simulink model "multi__micro1primarysecondarynn"  (R2015a)
settings: Solver=ode23tb  StartTime=0.0  StopTime=2
model workspace: external: MAT-File D:\google drive\project\nn1\matla.mat (data not in the file)
undefined symbols (not defined in the file): cf, gam, gamp, k1, k2, k3, k5, Lc, lf, mp1, mp2, Mu, nq1, nq2, rc, sig, sigp, td, wn
libraries: powerlib x115, powerlib_meascontrol x32, powerlib_extras x2
(part 2 of 3)

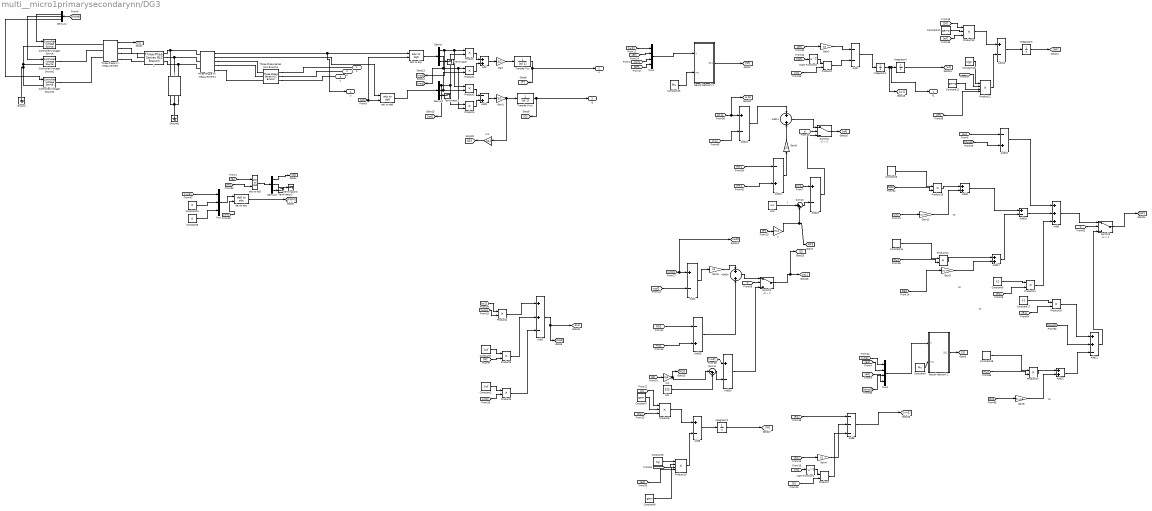
== system multi__micro1primarysecondarynn/DG3 ==
  note: SE
  note: SE
  note: SE
  note: SE
  Add{,3,11,14,17,22} (6 alike) : Sum
  Add{1,13,15..16} (4 alike) : Sum  Inputs=-+
  Add{4,9..10,12,18,20,23} (7 alike) : Sum  Inputs=+-
  Add2 : Sum  Inputs=++-
  Add21 : Sum  Inputs=++-
  Add5 : Sum  Inputs=+++
  Add7 : Sum  Inputs=--
  Add8 : Sum  Inputs=---
  C : powerlib/Elements/Three-Phase Series RLC Branch  LConnTagsString=A|B|C  RConnTagsString=A|B|C  BranchType=C  Resistance=1  Inductance=1e-3  Capacitance=cf  Measurements=None
  Constant1 : Constant  Value=1/cf
  Constant10 : Constant  Value=0
  Constant11 : Constant  Value=gamp
  Constant12 : Constant  Value=gamp
  Constant13 : Constant  Value=sigp
  Constant14 : Constant  Value=-31.446
  Constant15 : Constant  Value=Mu
  Constant17 : Constant  Value=k1
  Constant18 : Constant  Value=-31.446
  Constant2 : Constant  Value=1/cf
  Constant3 : Constant  Value=-31.446
  Constant4 : Constant  Value=Mu
  Constant5 : Constant  Value=k1
  Constant6 : Constant  Value=0
  Constant7 : Constant  Value=gam
  Constant8 : Constant  Value=sig
  Constant9 : Constant  Value=gam
  Controlled Voltage Source : powerlib/Electrical Sources/Controlled Voltage Source  Initialize=on  Source_Type=AC  Amplitude=0  Phase=0  Frequency=0  Measurements=None
  Controlled Voltage Source1 : powerlib/Electrical Sources/Controlled Voltage Source  Initialize=on  Source_Type=AC  Amplitude=0  Phase=0  Frequency=0  Measurements=None
  Controlled Voltage Source2 : powerlib/Electrical Sources/Controlled Voltage Source  Initialize=on  Source_Type=AC  Amplitude=0  Phase=0  Frequency=0  Measurements=None
  Demux{,1,3..4} (4 alike) : Demux  Outputs=3
  Gain : Gain  Gain=3/2
  Gain1 : Gain  Gain=3/2
  Gain11 : Gain  Gain=31.446
  Gain2 : Gain  Gain=k3
  Gain3 : Gain  Gain=31.446
  Gain4 : Gain  Gain=k2
  Gain5 : Gain  Gain=k5
  Gain6 : Gain  Gain=k5
  Gain8 : Gain  Gain=31.446
  Ground : powerlib/Elements/Ground  LConnTagsString=a
  Ground1 : powerlib/Elements/Ground  LConnTagsString=a
  Integrator1 : Integrator  UpperSaturationLimit=321  LowerSaturationLimit=314.16
  Integrator2 : Integrator  InitialCondition=zeros(16,1)  UpperSaturationLimit=314.16  ZeroCross=off
  Integrator3 : Integrator  InitialCondition=zeros(16,1)  UpperSaturationLimit=314.16  ZeroCross=off
  Integrator4 : Integrator  UpperSaturationLimit=314.16  ZeroCross=off
  L : powerlib/Elements/Three-Phase Series RLC Branch  LConnTagsString=A|B|C  RConnTagsString=A|B|C  BranchType=RL  Resistance=0.1  Inductance=lf  Capacitance=1e-6  Measurements=None
  Math Function1 : Math  Operator=transpose  OutputSignalType=real  SaturateOnIntegerOverflow=on
  Math Function3 : Math  Operator=transpose  OutputSignalType=real  SaturateOnIntegerOverflow=on
  Mux : Mux  Inputs=3
  Mux1 : Mux
  Mux2 : Mux
  Neural Network 1 : MATLAB Function  TreatAsAtomicUnit=on
  Neural Network 2 : MATLAB Function  TreatAsAtomicUnit=on
  Product{,1,3..4} (4 alike) : Product  RndMeth=Zero
  Product10 : Product  Inputs=4
  Product{2,5..6,11,14..17} (8 alike) : Product
  Product12 : Product  Inputs=4
  Product13 : Product  Inputs=3
  Product7 : Product  Multiplication=Matrix(*)
  Product8 : Product  Inputs=3
  Product9 : Product  Multiplication=Matrix(*)
  Sum10 : Sum  Inputs=|+-
  Sum11 : Sum  Inputs=|-+
  Switch2 : Switch  Criteria=u2 > Threshold
  Switch3 : Switch  Criteria=u2 > Threshold
  Switch4 : Switch  Criteria=u2 > Threshold
  Terminator{,1..3} (4 alike) : Terminator
  Three-Phase Series RLC Branch4 : powerlib/Elements/Three-Phase Series RLC Branch  LConnTagsString=A|B|C  RConnTagsString=A|B|C  BranchType=RL  Resistance=rc  Inductance=Lc  Capacitance=1e-6  Measurements=None
  Three-Phase V-I Measurement : powerlib/Measurements/Three-Phase V-I Measurement  VoltageMeasurement=no  SetLabelV=off  LabelV=Vabc  Vpu=off  VpuLL=off  CurrentMeasurement=yes  SetLabelI=off  LabelI=Iabc  Ipu=off  Pbase=100e6  Vbase=500e3  OutputType=Complex  PhasorSimulation=off  PSBequivalent=0
  Three-Phase V-I Measurement1 : powerlib/Measurements/Three-Phase V-I Measurement  VoltageMeasurement=phase-to-ground  SetLabelV=off  LabelV=Vabc  Vpu=off  VpuLL=off  CurrentMeasurement=yes  SetLabelI=off  LabelI=Iabc  Ipu=off  Pbase=100e6  Vbase=500e3  OutputType=Complex  PhasorSimulation=off  PSBequivalent=0
  Transfer Fcn : TransferFcn  Denominator=[td 1]
  Transfer Fcn1 : TransferFcn  Denominator=[td 1]
  Un1 : Constant  Value=325
  Un3 : Constant  Value=wn
  abc to dq0 : powerlib_meascontrol/Transformations/abc to dq0  Alignment=90 degrees behind phase A axis
  abc to dq1 : powerlib_meascontrol/Transformations/abc to dq0  Alignment=90 degrees behind phase A axis
  abc to dq3 : powerlib_meascontrol/Transformations/abc to dq0  Alignment=90 degrees behind phase A axis
  dq0 to abc : powerlib_meascontrol/Transformations/dq0 to abc  Alignment=90 degrees behind phase A axis
  m1 : Gain  Gain=nq1
  m2 : Gain  Gain=nq1
  n : Gain  Gain=mp1
  a : PMIOPort  Tag=PMCPort  Port=1  Side=Right
  b : PMIOPort  Tag=PMCPort  Port=2  Side=Right
  c : PMIOPort  Tag=PMCPort  Port=3  Side=Right
  U : Outport
  P : Outport  Port=2
  Q : Outport  Port=3
  f1 : Outport  Port=4
  tag scope: E3=global, MP3=global, NQ3=global, Q33=global, dv3=global, vod3=global, w13=global
  wires:
  [PWM] -> Demux4/1
  Three-Phase V-I Measurement1/1 -> U/1, abc to dq1/1
  Three-Phase V-I Measurement1/2 -> abc to dq0/1
  Demux/1 -> [vod], Product/1, Product3/1
  Demux1/1 -> [iod], Product/2, Product4/1
  Demux/2 -> [voq], Product1/1, Product4/2
  Demux1/2 -> Product1/2, Product3/2
  Product/1 -> Add/1
  Product1/1 -> Add/2
  Product3/1 -> Add1/1
  Product4/1 -> Add1/2
  [wt] -> abc to dq1/2, abc to dq0/2
  Demux4/1 -> Controlled Voltage Source/1
  Demux4/2 -> Controlled Voltage Source1/1
  Demux4/3 -> Controlled Voltage Source2/1
  Three-Phase V-I Measurement/1 -> [IL]
  Add/1 -> Gain/1
  Gain/1 -> Transfer Fcn/1
  Add1/1 -> Gain1/1
  Gain1/1 -> m1/1, Transfer Fcn1/1
  abc to dq1/1 -> Demux/1
  abc to dq0/1 -> Demux1/1
  [w1] -> Product2/1
  [voq] -> Product2/2
  Product2/1 -> Add2/1
  Constant1/1 -> Product5/1
  [Id] -> Product5/2
  Product5/1 -> Add2/2
  Constant2/1 -> Product6/1
  [iod] -> Product6/2
  Product6/1 -> Add2/3
  Add2/1 -> [dvodi], [dv3]
  Demux/3 -> Terminator/1
  Demux1/3 -> Terminator1/1
  Gain4/1 -> Add8/2
  [e2] -> Gain4/1
  [S] -> Product7/2
  [W] -> Math Function1/1
  Math Function1/1 -> Product7/1
  Product7/1 -> Add8/3
  Add8/1 -> [vn1]
  [IL] -> abc to dq3/1
  Demux3/1 -> [Id]
  Demux3/2 -> Terminator3/1
  [wt] -> abc to dq3/2
  Mux/1 -> dq0 to abc/1
  [wt] -> dq0 to abc/2
  abc to dq3/1 -> Demux3/1
  dq0 to abc/1 -> [PWM]
  Demux3/3 -> Terminator2/1
  [vn1] -> Mux/1
  Constant10/1 -> Mux/2
  Constant6/1 -> Mux/3
  Transfer Fcn/1 -> P/1, [P]
  Transfer Fcn1/1 -> Q/1, [Q]
  [ef] -> Gain2/1
  [Sf] -> Product9/2
  [Wf] -> Math Function3/1
  Math Function3/1 -> Product9/1
  Gain2/1 -> Add7/1
  Product9/1 -> Add7/2
  [w1] -> Mux1/1
  [ef] -> Mux1/2
  [wn] -> Mux1/3
  [MP1] -> Mux1/4
  [w1] -> [w13], Add10/1
  [w12] -> Add10/2
  Add10/1 -> Add11/1
  [MP1] -> Add13/1
  [MP3] -> Add13/2
  Add13/1 -> Gain6/1
  [vod] -> [vod3], Add4/1
  [vod2] -> Add4/2
  Add4/1 -> Gain5/1
  Add15/1 -> Add14/2
  Gain6/1 -> Add11/2
  [NQ1] -> Add15/1
  [NQ3] -> Add15/2
  [e1] -> Add8/1
  Gain5/1 -> Add14/1
  [vod] -> Mux2/1
  [e1] -> Mux2/2
  [e2] -> Mux2/4
  [dvodi] -> Mux2/3
  Constant3/1 -> Product15/1
  [NQ3] -> Product15/2
  Product15/1 -> Add3/1
  [Q33] -> Gain11/1
  Constant14/1 -> Product14/1
  [NQ1] -> Product14/2
  Product14/1 -> Add17/1
  [Q22] -> Gain3/1
  Add17/1 -> Add18/2
  Add3/1 -> Add18/1
  Gain3/1 -> Add17/2
  Gain11/1 -> Add3/2
  Add18/1 -> Add5/2
  Constant5/1 -> Product11/1
  [e1] -> Product11/2
  Product11/1 -> Add5/3
  [dv2] -> Add16/1
  Add16/1 -> Add5/1
  [dvodi] -> Add16/2
  m1/1 -> [Q33]
  Neural Network 1/1(Sz1) -> [Sf]
  Neural Network 2/1(Sz1) -> [S]
  [S] -> Product8/1
  Constant7/1 -> Product8/2
  [e2] -> Product8/3
  Product8/1 -> Add9/1
  Constant8/1 -> Product10/1
  [W] -> Product10/2
  Product10/1 -> Add9/2
  Constant9/1 -> Product10/3
  Add9/1 -> Integrator2/1
  Integrator2/1 -> [W]
  [e2] -> Product10/4
  [Sf] -> Product13/1
  Constant12/1 -> Product13/2
  [ef] -> Product13/3
  Product13/1 -> Add12/1
  Constant13/1 -> Product12/1
  [Wf] -> Product12/2
  Product12/1 -> Add12/2
  Constant11/1 -> Product12/3
  Add12/1 -> Integrator3/1
  Integrator3/1 -> [Wf]
  [ef] -> Product12/4
  Constant4/1 -> Neural Network 2/2(mu)
  Mux2/1 -> Neural Network 2/1(X)
  Constant15/1 -> Neural Network 1/2(mu)
  Mux1/1 -> Neural Network 1/1(X)
  [ti] -> Switch2/2
  Add20/1 -> Switch2/3
  Add14/1 -> Switch2/1
  Switch2/1 -> [E3], [e1]
  [vod] -> Add20/1
  [Q] -> m2/1
  Un1/1 -> Sum11/2
  m2/1 -> [NQ3], Sum11/1
  Sum11/1 -> Add20/2
  [dvodi] -> Add21/2
  Constant17/1 -> Product16/1
  [e1] -> Product16/2
  Product16/1 -> Add21/1
  Constant18/1 -> Product17/1
  [NQ3] -> Product17/2
  Product17/1 -> Add22/1
  [Q33] -> Gain8/1
  Add22/1 -> Add21/3
  Gain8/1 -> Add22/2
  [ti] -> Switch3/2
  Add5/1 -> Switch3/1
  Switch3/1 -> [e2]
  Add21/1 -> Switch3/3
  [P] -> n/1
  Un3/1 -> Sum10/1  "f"
  Sum10/1 -> Add23/2
  n/1 -> [MP3], Sum10/2
  [w1] -> Add23/1
  [ti] -> Switch4/2
  Add11/1 -> Switch4/1
  Switch4/1 -> [ef]
  Add23/1 -> Switch4/3
  Add7/1 -> Integrator1/1
  Integrator4/1 -> [wt]
  Integrator1/1 -> [w1], f1/1, Integrator4/1
  connections:
  C/RConn1 -- Ground1/LConn1 -- C/RConn3 -- C/RConn2
  L/RConn2 -- Three-Phase V-I Measurement1/LConn2 -- C/LConn2
  L/RConn1 -- Three-Phase V-I Measurement1/LConn1 -- C/LConn1
  L/RConn3 -- Three-Phase V-I Measurement1/LConn3 -- C/LConn3
  Controlled Voltage Source/LConn1 -- Controlled Voltage Source1/LConn1 -- Ground/LConn1 -- Controlled Voltage Source2/LConn1
  Three-Phase V-I Measurement/LConn1 -- Controlled Voltage Source/RConn1
  Controlled Voltage Source1/RConn1 -- Three-Phase V-I Measurement/LConn2
  Controlled Voltage Source2/RConn1 -- Three-Phase V-I Measurement/LConn3
  Three-Phase V-I Measurement/RConn1 -- L/LConn1
  Three-Phase V-I Measurement/RConn2 -- L/LConn2
  Three-Phase V-I Measurement/RConn3 -- L/LConn3
  Three-Phase V-I Measurement1/RConn1 -- Three-Phase Series RLC Branch4/RConn1
  Three-Phase V-I Measurement1/RConn2 -- Three-Phase Series RLC Branch4/RConn2
  Three-Phase V-I Measurement1/RConn3 -- Three-Phase Series RLC Branch4/RConn3
  Three-Phase Series RLC Branch4/LConn1 -- a/RConn1
  Three-Phase Series RLC Branch4/LConn2 -- b/RConn1
  Three-Phase Series RLC Branch4/LConn3 -- c/RConn1

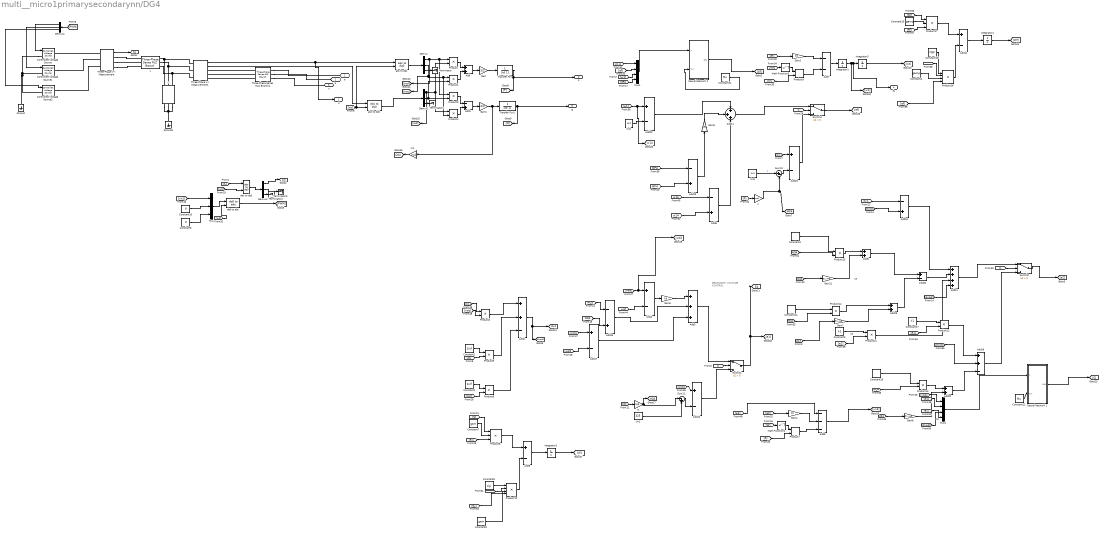
== system multi__micro1primarysecondarynn/DG4 ==
  note: SECONDARY VOLTAGE CONTROL
  note: SE
  note: SE
  note: SE
  Add{,5,19,22} (4 alike) : Sum
  Add{1,6,13,15,18} (5 alike) : Sum  Inputs=-+
  Add{4,9..10,12,14,17,20,23} (8 alike) : Sum  Inputs=+-
  Add11 : Sum  Inputs=+++
  Add16 : Sum  Inputs=++-
  Add2 : Sum  Inputs=++-
  Add21 : Sum  Inputs=++++
  Add3 : Sum  Inputs=+++
  Add7 : Sum  Inputs=--
  Add8 : Sum  Inputs=---
  C : powerlib/Elements/Three-Phase Series RLC Branch  LConnTagsString=A|B|C  RConnTagsString=A|B|C  BranchType=C  Resistance=1  Inductance=1e-3  Capacitance=cf  Measurements=None
  Constant1 : Constant  Value=1/cf
  Constant10 : Constant  Value=0
  Constant11 : Constant  Value=Mu
  Constant12 : Constant  Value=Mu
  Constant14 : Constant  Value=-31.446
  Constant15 : Constant  Value=gamp
  Constant16 : Constant  Value=sigp
  Constant17 : Constant  Value=k1
  Constant18 : Constant  Value=-31.446
  Constant2 : Constant  Value=1/cf
  Constant3 : Constant  Value=-31.446
  Constant4 : Constant  Value=gamp
  Constant5 : Constant  Value=k1
  Constant6 : Constant  Value=0
  Constant7 : Constant  Value=gam
  Constant8 : Constant  Value=sig
  Constant9 : Constant  Value=gam
  Controlled Voltage Source : powerlib/Electrical Sources/Controlled Voltage Source  Initialize=off  Source_Type=AC  Amplitude=325  Phase=0  Frequency=50  Measurements=None
  Controlled Voltage Source1 : powerlib/Electrical Sources/Controlled Voltage Source  Initialize=off  Source_Type=AC  Amplitude=325  Phase=0  Frequency=50  Measurements=None
  Controlled Voltage Source2 : powerlib/Electrical Sources/Controlled Voltage Source  Initialize=off  Source_Type=AC  Amplitude=325  Phase=0  Frequency=50  Measurements=None
  Demux{,1,3..4} (4 alike) : Demux  Outputs=3
  Gain : Gain  Gain=3/2
  Gain1 : Gain  Gain=3/2
  Gain11 : Gain  Gain=31.446
  Gain2 : Gain  Gain=k3
  Gain4 : Gain  Gain=k2
  Gain5 : Gain  Gain=k5
  Gain6 : Gain  Gain=k5
  Gain7 : Gain  Gain=31.446
  Gain8 : Gain  Gain=31.446
  Ground : powerlib/Elements/Ground  LConnTagsString=a
  Ground1 : powerlib/Elements/Ground  LConnTagsString=a
  Integrator1 : Integrator  UpperSaturationLimit=321  LowerSaturationLimit=314.16
  Integrator2 : Integrator  InitialCondition=zeros(16,1)  UpperSaturationLimit=314.16  ZeroCross=off
  Integrator3 : Integrator  UpperSaturationLimit=314.16  ZeroCross=off
  Integrator4 : Integrator  InitialCondition=zeros(16,1)  UpperSaturationLimit=314.16  ZeroCross=off
  L : powerlib/Elements/Three-Phase Series RLC Branch  LConnTagsString=A|B|C  RConnTagsString=A|B|C  BranchType=RL  Resistance=0.1  Inductance=lf  Capacitance=1e-6  Measurements=None
  Math Function1 : Math  Operator=transpose  OutputSignalType=real  SaturateOnIntegerOverflow=on
  Math Function3 : Math  Operator=transpose  OutputSignalType=real  SaturateOnIntegerOverflow=on
  Mux : Mux  Inputs=3
  Mux1 : Mux
  Mux2 : Mux
  Neural Network 1 : MATLAB Function  TreatAsAtomicUnit=on
  Neural Network 2 : MATLAB Function  TreatAsAtomicUnit=on
  Product{,1,3..4} (4 alike) : Product  RndMeth=Zero
  Product10 : Product  Inputs=4
  Product{2,5..6,11..15} (8 alike) : Product
  Product16 : Product  Inputs=4
  Product17 : Product  Inputs=3
  Product7 : Product  Multiplication=Matrix(*)
  Product8 : Product  Inputs=3
  Product9 : Product  Multiplication=Matrix(*)
  Sum10 : Sum  Inputs=|+-
  Sum11 : Sum  Inputs=|-+
  Switch2 : Switch  Criteria=u2 > Threshold
  Switch3 : Switch  Criteria=u2 > Threshold
  Switch4 : Switch  Criteria=u2 > Threshold
  Terminator{,1..3} (4 alike) : Terminator
  Three-Phase Series RLC Branch4 : powerlib/Elements/Three-Phase Series RLC Branch  LConnTagsString=A|B|C  RConnTagsString=A|B|C  BranchType=RL  Resistance=rc  Inductance=Lc  Capacitance=1e-6  Measurements=None
  Three-Phase V-I Measurement : powerlib/Measurements/Three-Phase V-I Measurement  VoltageMeasurement=no  SetLabelV=off  LabelV=Vabc  Vpu=off  VpuLL=off  CurrentMeasurement=yes  SetLabelI=off  LabelI=Iabc  Ipu=off  Pbase=100e6  Vbase=500e3  OutputType=Complex  PhasorSimulation=off  PSBequivalent=0
  Three-Phase V-I Measurement1 : powerlib/Measurements/Three-Phase V-I Measurement  VoltageMeasurement=phase-to-ground  SetLabelV=off  LabelV=Vabc  Vpu=off  VpuLL=off  CurrentMeasurement=yes  SetLabelI=off  LabelI=Iabc  Ipu=off  Pbase=100e6  Vbase=500e3  OutputType=Complex  PhasorSimulation=off  PSBequivalent=0
  Transfer Fcn : TransferFcn  Denominator=[td 1]
  Transfer Fcn1 : TransferFcn  Denominator=[td 1]
  Un1 : Constant  Value=325
  Un2 : Constant  Value=wn
  Un3 : Constant  Value=wn
  abc to dq0 : powerlib_meascontrol/Transformations/abc to dq0  Alignment=90 degrees behind phase A axis
  abc to dq1 : powerlib_meascontrol/Transformations/abc to dq0  Alignment=90 degrees behind phase A axis
  abc to dq3 : powerlib_meascontrol/Transformations/abc to dq0  Alignment=90 degrees behind phase A axis
  dq0 to abc : powerlib_meascontrol/Transformations/dq0 to abc  Alignment=90 degrees behind phase A axis
  m : Gain  Gain=nq1
  m1 : Gain  Gain=nq1
  n : Gain  Gain=mp1
  a : PMIOPort  Tag=PMCPort  Port=1  Side=Right
  b : PMIOPort  Tag=PMCPort  Port=2  Side=Right
  c : PMIOPort  Tag=PMCPort  Port=3  Side=Right
  U : Outport
  P : Outport  Port=2
  Q : Outport  Port=3
  f1 : Outport  Port=4
  tag scope: E4=global, MP4=global, NQ4=global, Q44=global, dv4=global, vod4=global, w14=global
  wires:
  [PWM] -> Demux4/1
  Three-Phase V-I Measurement1/1 -> U/1, abc to dq1/1
  Demux/1 -> [vod], Product/1, Product3/1
  Demux1/1 -> [iod], Product/2, Product4/1
  Demux/2 -> [voq], Product1/1, Product4/2
  Demux1/2 -> Product1/2, Product3/2
  Product/1 -> Add/1
  Product1/1 -> Add/2
  Product3/1 -> Add1/1
  Product4/1 -> Add1/2
  [wt] -> abc to dq1/2, abc to dq0/2
  Demux4/1 -> Controlled Voltage Source/1
  Demux4/2 -> Controlled Voltage Source1/1
  Demux4/3 -> Controlled Voltage Source2/1
  Three-Phase V-I Measurement/1 -> [IL]
  Add/1 -> Gain/1
  Gain/1 -> Transfer Fcn/1
  Add1/1 -> Gain1/1
  Gain1/1 -> m1/1, Transfer Fcn1/1
  abc to dq1/1 -> Demux/1
  abc to dq0/1 -> Demux1/1
  [w1] -> Product2/1
  [voq] -> Product2/2
  Product2/1 -> Add2/1
  Constant1/1 -> Product5/1
  [Id] -> Product5/2
  Product5/1 -> Add2/2
  Constant2/1 -> Product6/1
  [iod] -> Product6/2
  Product6/1 -> Add2/3
  Add2/1 -> [dvodi], [dv4]
  Demux/3 -> Terminator/1
  Demux1/3 -> Terminator1/1
  [vod] -> [vod4], Add4/1
  Gain4/1 -> Add8/2
  [e2] -> Gain4/1
  [S] -> Product7/2
  [W] -> Math Function1/1
  Math Function1/1 -> Product7/1
  Product7/1 -> Add8/3
  [vref] -> Add4/2
  Add8/1 -> [vn1]
  [IL] -> abc to dq3/1
  Demux3/1 -> [Id]
  Demux3/2 -> Terminator3/1
  [wt] -> abc to dq3/2
  Mux/1 -> dq0 to abc/1
  [wt] -> dq0 to abc/2
  abc to dq3/1 -> Demux3/1
  dq0 to abc/1 -> [PWM]
  Demux3/3 -> Terminator2/1
  [vn1] -> Mux/1
  Constant10/1 -> Mux/2
  Constant6/1 -> Mux/3
  Transfer Fcn/1 -> P/1, [P]
  Transfer Fcn1/1 -> Q/1, [Q]
  [w1] -> Mux1/1
  [ef] -> Mux1/2
  [w1] -> Mux1/3
  [MP2] -> Mux1/4
  [ef] -> Gain2/1
  [Sf] -> Product9/2
  [Wf] -> Math Function3/1
  Math Function3/1 -> Product9/1
  Gain2/1 -> Add7/1
  Product9/1 -> Add7/2
  [w1] -> [w14], Add10/1
  Un2/1 -> Add10/2
  Add10/1 -> Add11/1
  Three-Phase V-I Measurement1/2 -> abc to dq0/1
  [MP3] -> Add13/1
  [MP4] -> Add13/2
  Add13/1 -> Gain6/1
  Gain6/1 -> Add11/2
  [NQ3] -> Add15/1
  [NQ4] -> Add15/2
  [e1] -> Add8/1
  Add4/1 -> Gain5/1
  Gain5/1 -> Add3/1
  Add15/1 -> Add3/2
  [vod3] -> Add17/2
  [vod] -> Add17/1
  Add17/1 -> Add3/3
  Constant3/1 -> Product15/1
  [NQ4] -> Product15/2
  Product15/1 -> Add5/1
  [Q44] -> Gain11/1
  Constant14/1 -> Product14/1
  [NQ3] -> Product14/2
  Product14/1 -> Add19/1
  [Q33] -> Gain7/1
  Add19/1 -> Add20/2
  Add5/1 -> Add20/1
  Gain7/1 -> Add19/2
  Gain11/1 -> Add5/2
  Add20/1 -> Add21/2
  Constant5/1 -> Product11/1
  [e1] -> Product11/2
  Product11/1 -> Add21/3
  [dv3] -> Add18/1
  Add18/1 -> Add21/1
  [dvodi] -> Add18/2
  [vod] -> Mux2/1
  [e1] -> Mux2/2
  [e2] -> Mux2/4
  [dvodi] -> Mux2/3
  [dvodi] -> Add21/4
  m1/1 -> [Q44]
  [w13] -> Add6/1
  [w14] -> Add6/2
  Add6/1 -> Add11/3
  [S] -> Product8/1
  Constant7/1 -> Product8/2
  [e2] -> Product8/3
  Product8/1 -> Add9/1
  Constant8/1 -> Product10/1
  [W] -> Product10/2
  Product10/1 -> Add9/2
  Constant9/1 -> Product10/3
  Add9/1 -> Integrator2/1
  Integrator2/1 -> [W]
  [e2] -> Product10/4
  [Sf] -> Product17/1
  Constant15/1 -> Product17/2
  [ef] -> Product17/3
  Product17/1 -> Add14/1
  Constant16/1 -> Product16/1
  [Wf] -> Product16/2
  Product16/1 -> Add14/2
  Constant4/1 -> Product16/3
  Add14/1 -> Integrator4/1
  Integrator4/1 -> [Wf]
  [ef] -> Product16/4
  Neural Network 2/1(Sz1) -> [Sf]
  Constant11/1 -> Neural Network 2/2(mu)
  Mux1/1 -> Neural Network 2/1(X)
  Neural Network 1/1(Sz1) -> [S]
  Constant12/1 -> Neural Network 1/2(mu)
  Mux2/1 -> Neural Network 1/1(X)
  [vod] -> Add12/1
  [Q] -> m/1
  Un1/1 -> Sum11/2
  m/1 -> [NQ4], Sum11/1
  Sum11/1 -> Add12/2
  [ti] -> Switch2/2
  Add12/1 -> Switch2/3
  Add3/1 -> Switch2/1
  Switch2/1 -> [E4], [e1]
  [dvodi] -> Add16/2
  Constant17/1 -> Product12/1
  [e1] -> Product12/2
  Product12/1 -> Add16/1
  Constant18/1 -> Product13/1
  [NQ4] -> Product13/2
  Product13/1 -> Add22/1
  [Q44] -> Gain8/1
  Add22/1 -> Add16/3
  Gain8/1 -> Add22/2
  [ti] -> Switch3/2
  Switch3/1 -> [e2]
  Add21/1 -> Switch3/1
  Add16/1 -> Switch3/3
  Add7/1 -> Integrator1/1
  Integrator3/1 -> [wt]
  Integrator1/1 -> [w1], f1/1, Integrator3/1
  [ti] -> Switch4/2
  Add11/1 -> Switch4/1
  Switch4/1 -> [ef]
  [P] -> n/1
  Un3/1 -> Sum10/1  "f"
  Sum10/1 -> Add23/2
  n/1 -> [MP4], Sum10/2
  [w1] -> Add23/1
  Add23/1 -> Switch4/3
  connections:
  C/RConn1 -- Ground1/LConn1 -- C/RConn3 -- C/RConn2
  L/RConn2 -- Three-Phase V-I Measurement1/LConn2 -- C/LConn2
  L/RConn1 -- Three-Phase V-I Measurement1/LConn1 -- C/LConn1
  L/RConn3 -- Three-Phase V-I Measurement1/LConn3 -- C/LConn3
  Controlled Voltage Source/LConn1 -- Controlled Voltage Source1/LConn1 -- Ground/LConn1 -- Controlled Voltage Source2/LConn1
  Three-Phase V-I Measurement/LConn1 -- Controlled Voltage Source/RConn1
  Controlled Voltage Source1/RConn1 -- Three-Phase V-I Measurement/LConn2
  Controlled Voltage Source2/RConn1 -- Three-Phase V-I Measurement/LConn3
  Three-Phase V-I Measurement/RConn1 -- L/LConn1
  Three-Phase V-I Measurement/RConn2 -- L/LConn2
  Three-Phase V-I Measurement/RConn3 -- L/LConn3
  Three-Phase Series RLC Branch4/RConn1 -- Three-Phase V-I Measurement1/RConn1
  Three-Phase Series RLC Branch4/RConn2 -- Three-Phase V-I Measurement1/RConn2
  Three-Phase Series RLC Branch4/RConn3 -- Three-Phase V-I Measurement1/RConn3
  Three-Phase Series RLC Branch4/LConn3 -- c/RConn1
  Three-Phase Series RLC Branch4/LConn2 -- b/RConn1
  Three-Phase Series RLC Branch4/LConn1 -- a/RConn1

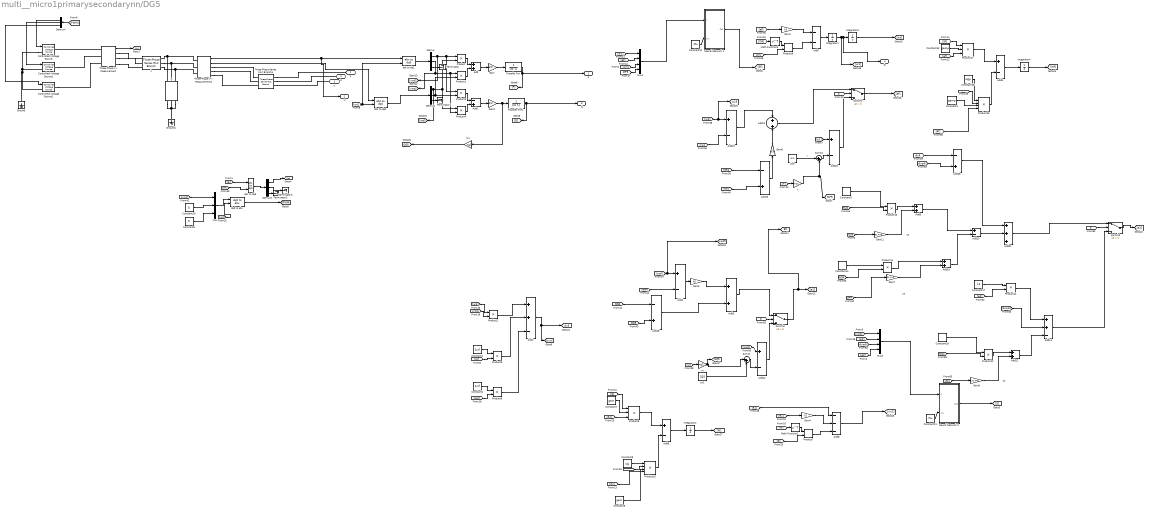
== system multi__micro1primarysecondarynn/DG5 ==
  note: SE
  note: SE
  note: SE
  Add{,3,5,11,19,22} (6 alike) : Sum
  Add{1,13,15,18} (4 alike) : Sum  Inputs=-+
  Add{4,6,9..10,12,20,23} (7 alike) : Sum  Inputs=+-
  Add14 : Sum  Inputs=++-
  Add2 : Sum  Inputs=++-
  Add21 : Sum  Inputs=+++
  Add7 : Sum  Inputs=--
  Add8 : Sum  Inputs=---
  C : powerlib/Elements/Three-Phase Series RLC Branch  LConnTagsString=A|B|C  RConnTagsString=A|B|C  BranchType=C  Resistance=1  Inductance=1e-3  Capacitance=cf  Measurements=None
  Constant1 : Constant  Value=1/cf
  Constant10 : Constant  Value=0
  Constant11 : Constant  Value=Mu
  Constant12 : Constant  Value=Mu
  Constant14 : Constant  Value=-31.446
  Constant15 : Constant  Value=gamp
  Constant16 : Constant  Value=sigp
  Constant17 : Constant  Value=k1
  Constant18 : Constant  Value=-31.446
  Constant2 : Constant  Value=1/cf
  Constant3 : Constant  Value=-31.446
  Constant4 : Constant  Value=gamp
  Constant6 : Constant  Value=0
  Constant7 : Constant  Value=gam
  Constant8 : Constant  Value=sig
  Constant9 : Constant  Value=gam
  Controlled Voltage Source : powerlib/Electrical Sources/Controlled Voltage Source  Initialize=off  Source_Type=AC  Amplitude=325  Phase=0  Frequency=50  Measurements=None
  Controlled Voltage Source1 : powerlib/Electrical Sources/Controlled Voltage Source  Initialize=off  Source_Type=AC  Amplitude=325  Phase=0  Frequency=50  Measurements=None
  Controlled Voltage Source2 : powerlib/Electrical Sources/Controlled Voltage Source  Initialize=off  Source_Type=AC  Amplitude=325  Phase=0  Frequency=50  Measurements=None
  Demux{,1,3..4} (4 alike) : Demux  Outputs=3
  Gain : Gain  Gain=3/2
  Gain1 : Gain  Gain=3/2
  Gain11 : Gain  Gain=31.446
  Gain2 : Gain  Gain=k3
  Gain4 : Gain  Gain=k2
  Gain5 : Gain  Gain=k5
  Gain6 : Gain  Gain=k5
  Gain7 : Gain  Gain=31.446
  Gain8 : Gain  Gain=31.446
  Ground : powerlib/Elements/Ground  LConnTagsString=a
  Ground1 : powerlib/Elements/Ground  LConnTagsString=a
  Integrator1 : Integrator  UpperSaturationLimit=321  LowerSaturationLimit=314.16
  Integrator2 : Integrator  InitialCondition=zeros(16,1)  UpperSaturationLimit=314.16  ZeroCross=off
  Integrator3 : Integrator  UpperSaturationLimit=314.16  ZeroCross=off
  Integrator4 : Integrator  InitialCondition=zeros(16,1)  UpperSaturationLimit=314.16  ZeroCross=off
  L : powerlib/Elements/Three-Phase Series RLC Branch  LConnTagsString=A|B|C  RConnTagsString=A|B|C  BranchType=RL  Resistance=0.1  Inductance=lf  Capacitance=1e-6  Measurements=None
  Math Function1 : Math  Operator=transpose  OutputSignalType=real  SaturateOnIntegerOverflow=on
  Math Function3 : Math  Operator=transpose  OutputSignalType=real  SaturateOnIntegerOverflow=on
  Mux : Mux  Inputs=3
  Mux1 : Mux
  Mux2 : Mux
  Neural Network 1 : MATLAB Function  TreatAsAtomicUnit=on
  Neural Network 2 : MATLAB Function  TreatAsAtomicUnit=on
  Product{,1,3..4} (4 alike) : Product  RndMeth=Zero
  Product10 : Product  Inputs=4
  Product{2,5..6,11..12,14..15} (7 alike) : Product
  Product16 : Product  Inputs=4
  Product17 : Product  Inputs=3
  Product7 : Product  Multiplication=Matrix(*)
  Product8 : Product  Inputs=3
  Product9 : Product  Multiplication=Matrix(*)
  Sum10 : Sum  Inputs=|+-
  Sum11 : Sum  Inputs=|-+
  Switch2 : Switch  Criteria=u2 > Threshold
  Switch3 : Switch  Criteria=u2 > Threshold
  Switch4 : Switch  Criteria=u2 > Threshold
  Terminator{,1..3} (4 alike) : Terminator
  Three-Phase Series RLC Branch4 : powerlib/Elements/Three-Phase Series RLC Branch  LConnTagsString=A|B|C  RConnTagsString=A|B|C  BranchType=RL  Resistance=rc  Inductance=Lc  Capacitance=1e-6  Measurements=None
  Three-Phase V-I Measurement : powerlib/Measurements/Three-Phase V-I Measurement  VoltageMeasurement=no  SetLabelV=off  LabelV=Vabc  Vpu=off  VpuLL=off  CurrentMeasurement=yes  SetLabelI=off  LabelI=Iabc  Ipu=off  Pbase=100e6  Vbase=500e3  OutputType=Complex  PhasorSimulation=off  PSBequivalent=0
  Three-Phase V-I Measurement1 : powerlib/Measurements/Three-Phase V-I Measurement  VoltageMeasurement=phase-to-ground  SetLabelV=off  LabelV=Vabc  Vpu=off  VpuLL=off  CurrentMeasurement=yes  SetLabelI=off  LabelI=Iabc  Ipu=off  Pbase=100e6  Vbase=500e3  OutputType=Complex  PhasorSimulation=off  PSBequivalent=0
  Transfer Fcn : TransferFcn  Denominator=[td 1]
  Transfer Fcn1 : TransferFcn  Denominator=[td 1]
  Un1 : Constant  Value=325
  Un3 : Constant  Value=wn
  abc to dq0 : powerlib_meascontrol/Transformations/abc to dq0  Alignment=90 degrees behind phase A axis
  abc to dq1 : powerlib_meascontrol/Transformations/abc to dq0  Alignment=90 degrees behind phase A axis
  abc to dq3 : powerlib_meascontrol/Transformations/abc to dq0  Alignment=90 degrees behind phase A axis
  dq0 to abc : powerlib_meascontrol/Transformations/dq0 to abc  Alignment=90 degrees behind phase A axis
  m : Gain  Gain=nq1
  m1 : Gain  Gain=nq1
  n : Gain  Gain=mp1
  a : PMIOPort  Tag=PMCPort  Port=1  Side=Right
  b : PMIOPort  Tag=PMCPort  Port=2  Side=Right
  c : PMIOPort  Tag=PMCPort  Port=3  Side=Right
  U : Outport
  P : Outport  Port=2
  Q : Outport  Port=3
  f1 : Outport  Port=4
  tag scope: E5=global, MP5=global, NQ5=global, Q55=global, dv5=global, vod5=global, w15=global
  wires:
  [PWM] -> Demux4/1
  Three-Phase V-I Measurement1/1 -> U/1, abc to dq1/1
  Three-Phase V-I Measurement1/2 -> abc to dq0/1
  Demux/1 -> [vod], Product/1, Product3/1
  Demux1/1 -> [iod], Product/2, Product4/1
  Demux/2 -> [voq], Product1/1, Product4/2
  Demux1/2 -> Product1/2, Product3/2
  Product/1 -> Add/1
  Product1/1 -> Add/2
  Product3/1 -> Add1/1
  Product4/1 -> Add1/2
  [wt] -> abc to dq1/2, abc to dq0/2
  Demux4/1 -> Controlled Voltage Source/1
  Demux4/2 -> Controlled Voltage Source1/1
  Demux4/3 -> Controlled Voltage Source2/1
  Three-Phase V-I Measurement/1 -> [IL]
  Add/1 -> Gain/1
  Gain/1 -> Transfer Fcn/1
  Add1/1 -> Gain1/1
  Gain1/1 -> m1/1, Transfer Fcn1/1
  abc to dq1/1 -> Demux/1
  abc to dq0/1 -> Demux1/1
  [w1] -> Product2/1
  [voq] -> Product2/2
  Product2/1 -> Add2/1
  Constant1/1 -> Product5/1
  [Id] -> Product5/2
  Product5/1 -> Add2/2
  Constant2/1 -> Product6/1
  [iod] -> Product6/2
  Product6/1 -> Add2/3
  Add2/1 -> [dvodi], [dv5]
  Demux/3 -> Terminator/1
  Demux1/3 -> Terminator1/1
  Gain4/1 -> Add8/2
  [e2] -> Gain4/1
  [S] -> Product7/2
  [W] -> Math Function1/1
  Math Function1/1 -> Product7/1
  Product7/1 -> Add8/3
  Add8/1 -> [vn1]
  [IL] -> abc to dq3/1
  Demux3/1 -> [Id]
  Demux3/2 -> Terminator3/1
  [wt] -> abc to dq3/2
  Mux/1 -> dq0 to abc/1
  [wt] -> dq0 to abc/2
  abc to dq3/1 -> Demux3/1
  dq0 to abc/1 -> [PWM]
  Demux3/3 -> Terminator2/1
  [vn1] -> Mux/1
  Constant10/1 -> Mux/2
  Constant6/1 -> Mux/3
  Transfer Fcn/1 -> P/1, [P]
  Transfer Fcn1/1 -> Q/1, [Q]
  [ef] -> Gain2/1
  [Sf] -> Product9/2
  [Wf] -> Math Function3/1
  Math Function3/1 -> Product9/1
  Gain2/1 -> Add7/1
  Product9/1 -> Add7/2
  [w1] -> Mux1/1
  [ef] -> Mux1/2
  [wn] -> Mux1/3
  [MP5] -> Mux1/4
  [w1] -> [w15], Add10/1
  [w14] -> Add10/2
  Add10/1 -> Add11/1
  [MP4] -> Add13/1
  [MP5] -> Add13/2
  Add13/1 -> Gain6/1
  [vod] -> [vod5], Add4/1
  [vod4] -> Add4/2
  Gain6/1 -> Add11/2
  [NQ4] -> Add15/1
  [NQ5] -> Add15/2
  [e1] -> Add8/1
  Add4/1 -> Gain5/1
  Add15/1 -> Add3/2
  Gain5/1 -> Add3/1
  Constant3/1 -> Product15/1
  [NQ5] -> Product15/2
  Product15/1 -> Add5/1
  [Q55] -> Gain11/1
  Constant14/1 -> Product14/1
  [NQ4] -> Product14/2
  Product14/1 -> Add19/1
  [Q44] -> Gain7/1
  Add19/1 -> Add20/2
  Add5/1 -> Add20/1
  Gain7/1 -> Add19/2
  Gain11/1 -> Add5/2
  Add20/1 -> Add21/2
  [dv4] -> Add18/1
  Add18/1 -> Add21/1
  [dvodi] -> Add18/2
  [vod] -> Mux2/1
  [e1] -> Mux2/2
  [e2] -> Mux2/4
  [dvodi] -> Mux2/3
  m1/1 -> [Q55]
  Neural Network 2/1(Sz1) -> [S]
  Neural Network 1/1(Sz1) -> [Sf]
  [S] -> Product8/1
  Constant7/1 -> Product8/2
  [e2] -> Product8/3
  Product8/1 -> Add9/1
  Constant8/1 -> Product10/1
  [W] -> Product10/2
  Product10/1 -> Add9/2
  Constant9/1 -> Product10/3
  Add9/1 -> Integrator2/1
  Integrator2/1 -> [W]
  [e2] -> Product10/4
  [Sf] -> Product17/1
  Constant15/1 -> Product17/2
  [ef] -> Product17/3
  Product17/1 -> Add6/1
  Constant16/1 -> Product16/1
  [Wf] -> Product16/2
  Product16/1 -> Add6/2
  Constant4/1 -> Product16/3
  Add6/1 -> Integrator4/1
  Integrator4/1 -> [Wf]
  [ef] -> Product16/4
  Constant11/1 -> Neural Network 2/2(mu)
  Mux2/1 -> Neural Network 2/1(X)
  Constant12/1 -> Neural Network 1/2(mu)
  Mux1/1 -> Neural Network 1/1(X)
  [ti] -> Switch4/2
  Add11/1 -> Switch4/1
  Switch4/1 -> [ef]
  [P] -> n/1
  Un3/1 -> Sum10/1  "f"
  Sum10/1 -> Add23/2
  n/1 -> [MP5], Sum10/2
  [w1] -> Add23/1
  Add23/1 -> Switch4/3
  Add7/1 -> Integrator1/1
  Integrator3/1 -> [wt]
  Integrator1/1 -> [w1], f1/1, Integrator3/1
  [ti] -> Switch2/2
  Add12/1 -> Switch2/3
  Add3/1 -> Switch2/1
  Switch2/1 -> [E5], [e1]
  [vod] -> Add12/1
  [Q] -> m/1
  Un1/1 -> Sum11/2
  m/1 -> [NQ5], Sum11/1
  Sum11/1 -> Add12/2
  [dvodi] -> Add14/2
  Constant17/1 -> Product11/1
  [e1] -> Product11/2
  Product11/1 -> Add14/1
  Constant18/1 -> Product12/1
  [NQ5] -> Product12/2
  Product12/1 -> Add22/1
  [Q55] -> Gain8/1
  Add22/1 -> Add14/3
  Gain8/1 -> Add22/2
  [ti] -> Switch3/2
  Switch3/1 -> [e2]
  Add21/1 -> Switch3/1
  Add14/1 -> Switch3/3
  connections:
  C/RConn1 -- Ground1/LConn1 -- C/RConn3 -- C/RConn2
  L/RConn2 -- Three-Phase V-I Measurement1/LConn2 -- C/LConn2
  L/RConn1 -- Three-Phase V-I Measurement1/LConn1 -- C/LConn1
  L/RConn3 -- Three-Phase V-I Measurement1/LConn3 -- C/LConn3
  Controlled Voltage Source/LConn1 -- Controlled Voltage Source1/LConn1 -- Ground/LConn1 -- Controlled Voltage Source2/LConn1
  Three-Phase V-I Measurement/LConn1 -- Controlled Voltage Source/RConn1
  Controlled Voltage Source1/RConn1 -- Three-Phase V-I Measurement/LConn2
  Controlled Voltage Source2/RConn1 -- Three-Phase V-I Measurement/LConn3
  Three-Phase V-I Measurement/RConn1 -- L/LConn1
  Three-Phase V-I Measurement/RConn2 -- L/LConn2
  Three-Phase V-I Measurement/RConn3 -- L/LConn3
  Three-Phase V-I Measurement1/RConn1 -- Three-Phase Series RLC Branch4/RConn1
  Three-Phase V-I Measurement1/RConn2 -- Three-Phase Series RLC Branch4/RConn2
  Three-Phase V-I Measurement1/RConn3 -- Three-Phase Series RLC Branch4/RConn3
  Three-Phase Series RLC Branch4/LConn1 -- a/RConn1
  Three-Phase Series RLC Branch4/LConn2 -- b/RConn1
  Three-Phase Series RLC Branch4/LConn3 -- c/RConn1

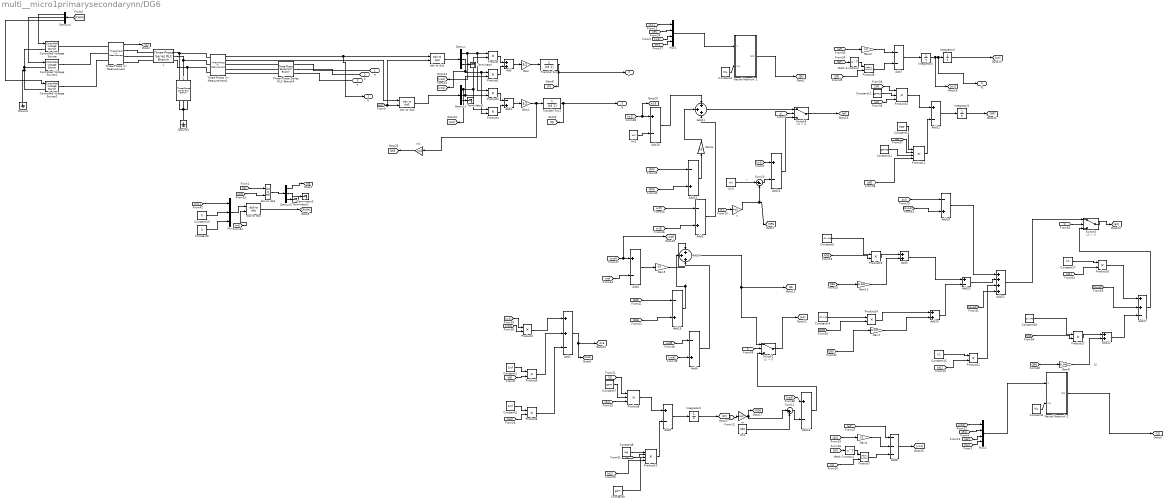
== system multi__micro1primarysecondarynn/DG6 ==
  note: SE
  Add{,5,19,22} (4 alike) : Sum
  Add{1,3,6,13,15,18} (6 alike) : Sum  Inputs=-+
  Add{4,9..10,12,16,20,23} (7 alike) : Sum  Inputs=+-
  Add11 : Sum  Inputs=+++
  Add14 : Sum  Inputs=+++
  Add17 : Sum  Inputs=++-
  Add2 : Sum  Inputs=++-
  Add21 : Sum  Inputs=++++
  Add7 : Sum  Inputs=--
  Add8 : Sum  Inputs=---
  C : powerlib/Elements/Three-Phase Series RLC Branch  LConnTagsString=A|B|C  RConnTagsString=A|B|C  BranchType=C  Resistance=1  Inductance=1e-3  Capacitance=cf  Measurements=None
  Constant1 : Constant  Value=1/cf
  Constant10 : Constant  Value=0
  Constant11 : Constant  Value=gamp
  Constant12 : Constant  Value=gamp
  Constant13 : Constant  Value=sigp
  Constant14 : Constant  Value=-31.446
  Constant15 : Constant  Value=k1
  Constant17 : Constant  Value=k1
  Constant18 : Constant  Value=-31.446
  Constant2 : Constant  Value=1/cf
  Constant3 : Constant  Value=Mu
  Constant4 : Constant  Value=Mu
  Constant5 : Constant  Value=-31.446
  Constant6 : Constant  Value=0
  Constant7 : Constant  Value=gam
  Constant8 : Constant  Value=sig
  Constant9 : Constant  Value=gam
  Controlled Voltage Source : powerlib/Electrical Sources/Controlled Voltage Source  Initialize=off  Source_Type=AC  Amplitude=325  Phase=0  Frequency=50  Measurements=None
  Controlled Voltage Source1 : powerlib/Electrical Sources/Controlled Voltage Source  Initialize=off  Source_Type=AC  Amplitude=325  Phase=0  Frequency=50  Measurements=None
  Controlled Voltage Source2 : powerlib/Electrical Sources/Controlled Voltage Source  Initialize=off  Source_Type=AC  Amplitude=325  Phase=0  Frequency=50  Measurements=None
  Demux{,1,3..4} (4 alike) : Demux  Outputs=3
  Gain : Gain  Gain=3/2
  Gain1 : Gain  Gain=3/2
  Gain11 : Gain  Gain=31.446
  Gain2 : Gain  Gain=k3
  Gain4 : Gain  Gain=k2
  Gain5 : Gain  Gain=k5
  Gain6 : Gain  Gain=k5
  Gain7 : Gain  Gain=31.446
  Gain8 : Gain  Gain=31.446
  Ground : powerlib/Elements/Ground  LConnTagsString=a
  Ground1 : powerlib/Elements/Ground  LConnTagsString=a
  Integrator1 : Integrator  UpperSaturationLimit=321  LowerSaturationLimit=314.16
  Integrator2 : Integrator  InitialCondition=zeros(16,1)  UpperSaturationLimit=314.16  ZeroCross=off
  Integrator3 : Integrator  InitialCondition=zeros(16,1)  UpperSaturationLimit=314.16  ZeroCross=off
  Integrator4 : Integrator  UpperSaturationLimit=314.16  ZeroCross=off
  L : powerlib/Elements/Three-Phase Series RLC Branch  LConnTagsString=A|B|C  RConnTagsString=A|B|C  BranchType=RL  Resistance=0.1  Inductance=lf  Capacitance=1e-6  Measurements=None
  Math Function1 : Math  Operator=transpose  OutputSignalType=real  SaturateOnIntegerOverflow=on
  Math Function3 : Math  Operator=transpose  OutputSignalType=real  SaturateOnIntegerOverflow=on
  Mux : Mux  Inputs=3
  Mux1 : Mux
  Mux2 : Mux
  Neural Network 1 : MATLAB Function  TreatAsAtomicUnit=on
  Neural Network 2 : MATLAB Function  TreatAsAtomicUnit=on
  Product{,1,3..4} (4 alike) : Product  RndMeth=Zero
  Product10 : Product  Inputs=4
  Product{2,5..6,11,14..17} (8 alike) : Product
  Product12 : Product  Inputs=4
  Product13 : Product  Inputs=3
  Product7 : Product  Multiplication=Matrix(*)
  Product8 : Product  Inputs=3
  Product9 : Product  Multiplication=Matrix(*)
  Sum10 : Sum  Inputs=|+-
  Sum11 : Sum  Inputs=|-+
  Switch2 : Switch  Criteria=u2 > Threshold
  Switch3 : Switch  Criteria=u2 > Threshold
  Switch4 : Switch  Criteria=u2 > Threshold
  Terminator{,1..3} (4 alike) : Terminator
  Three-Phase Series RLC Branch4 : powerlib/Elements/Three-Phase Series RLC Branch  LConnTagsString=A|B|C  RConnTagsString=A|B|C  BranchType=RL  Resistance=rc  Inductance=Lc  Capacitance=1e-6  Measurements=None
  Three-Phase V-I Measurement : powerlib/Measurements/Three-Phase V-I Measurement  VoltageMeasurement=no  SetLabelV=off  LabelV=Vabc  Vpu=off  VpuLL=off  CurrentMeasurement=yes  SetLabelI=off  LabelI=Iabc  Ipu=off  Pbase=100e6  Vbase=500e3  OutputType=Complex  PhasorSimulation=off  PSBequivalent=0
  Three-Phase V-I Measurement1 : powerlib/Measurements/Three-Phase V-I Measurement  VoltageMeasurement=phase-to-ground  SetLabelV=off  LabelV=Vabc  Vpu=off  VpuLL=off  CurrentMeasurement=yes  SetLabelI=off  LabelI=Iabc  Ipu=off  Pbase=100e6  Vbase=500e3  OutputType=Complex  PhasorSimulation=off  PSBequivalent=0
  Transfer Fcn : TransferFcn  Denominator=[td 1]
  Transfer Fcn1 : TransferFcn  Denominator=[td 1]
  Un1 : Constant  Value=325
  Un2 : Constant  Value=wn
  Un3 : Constant  Value=wn
  abc to dq0 : powerlib_meascontrol/Transformations/abc to dq0  Alignment=90 degrees behind phase A axis
  abc to dq1 : powerlib_meascontrol/Transformations/abc to dq0  Alignment=90 degrees behind phase A axis
  abc to dq3 : powerlib_meascontrol/Transformations/abc to dq0  Alignment=90 degrees behind phase A axis
  dq0 to abc : powerlib_meascontrol/Transformations/dq0 to abc  Alignment=90 degrees behind phase A axis
  m : Gain  Gain=nq2
  m1 : Gain  Gain=nq2
  n : Gain  Gain=mp2
  a : PMIOPort  Tag=PMCPort  Port=1  Side=Right
  b : PMIOPort  Tag=PMCPort  Port=2  Side=Right
  c : PMIOPort  Tag=PMCPort  Port=3  Side=Right
  U : Outport
  P : Outport  Port=2
  Q : Outport  Port=3
  f1 : Outport  Port=4
  tag scope: E6=global, MP6=global, NQ6=global, Q66=global, dv6=global, vod6=global, w16=global
  wires:
  [PWM] -> Demux4/1
  Three-Phase V-I Measurement1/1 -> U/1, abc to dq1/1
  Demux/1 -> [vod], Product/1, Product3/1
  Demux1/1 -> [iod], Product/2, Product4/1
  Demux/2 -> [voq], Product1/1, Product4/2
  Demux1/2 -> Product1/2, Product3/2
  Product/1 -> Add/1
  Product1/1 -> Add/2
  Product3/1 -> Add1/1
  Product4/1 -> Add1/2
  [wt] -> abc to dq1/2, abc to dq0/2
  Demux4/1 -> Controlled Voltage Source/1
  Demux4/2 -> Controlled Voltage Source1/1
  Demux4/3 -> Controlled Voltage Source2/1
  Three-Phase V-I Measurement/1 -> [IL]
  Add/1 -> Gain/1
  Gain/1 -> Transfer Fcn/1
  Add1/1 -> Gain1/1
  Gain1/1 -> m1/1, Transfer Fcn1/1
  abc to dq1/1 -> Demux/1
  abc to dq0/1 -> Demux1/1
  [w1] -> Product2/1
  [voq] -> Product2/2
  Product2/1 -> Add2/1
  Constant1/1 -> Product5/1
  [Id] -> Product5/2
  Product5/1 -> Add2/2
  Constant2/1 -> Product6/1
  [iod] -> Product6/2
  Product6/1 -> Add2/3
  Add2/1 -> [dvodi], [dv6]
  Demux/3 -> Terminator/1
  Demux1/3 -> Terminator1/1
  [vod] -> [vod6], Add4/1
  Gain4/1 -> Add8/2
  [e2] -> Gain4/1
  [S] -> Product7/2
  [W] -> Math Function1/1
  Math Function1/1 -> Product7/1
  Product7/1 -> Add8/3
  [vref] -> Add4/2
  [vod] -> Mux2/1
  [e1] -> Mux2/2
  [e2] -> Mux2/3
  [e2] -> Mux2/4
  [IL] -> abc to dq3/1
  Demux3/1 -> [Id]
  Demux3/2 -> Terminator3/1
  [wt] -> abc to dq3/2
  Mux/1 -> dq0 to abc/1
  [wt] -> dq0 to abc/2
  abc to dq3/1 -> Demux3/1
  dq0 to abc/1 -> [PWM]
  Demux3/3 -> Terminator2/1
  [vn1] -> Mux/1
  Constant10/1 -> Mux/2
  Constant6/1 -> Mux/3
  Transfer Fcn/1 -> P/1, [P]
  Transfer Fcn1/1 -> Q/1, [Q]
  [w1] -> Mux1/1
  [ef] -> Mux1/2
  [w1] -> Mux1/3
  [MP2] -> Mux1/4
  [ef] -> Gain2/1
  [Sf] -> Product9/2
  [Wf] -> Math Function3/1
  Math Function3/1 -> Product9/1
  Gain2/1 -> Add7/1
  Product9/1 -> Add7/2
  [w1] -> [w16], Add10/1
  Un2/1 -> Add10/2
  Add10/1 -> Add11/1
  Add4/1 -> Gain5/1
  Three-Phase V-I Measurement1/2 -> abc to dq0/1
  [NQ5] -> Add15/1
  [NQ6] -> Add15/2
  Add15/1 -> Add14/2
  [MP5] -> Add13/1
  [MP6] -> Add13/2
  Add13/1 -> Gain6/1
  Gain6/1 -> Add11/2
  [e1] -> Add8/1
  Add8/1 -> [vn1]
  m1/1 -> [Q66]
  Constant5/1 -> Product15/1
  [NQ6] -> Product15/2
  Product15/1 -> Add5/1
  [Q66] -> Gain11/1
  Constant14/1 -> Product14/1
  [NQ5] -> Product14/2
  Product14/1 -> Add19/1
  [Q55] -> Gain7/1
  Add19/1 -> Add20/2
  Add5/1 -> Add20/1
  Gain7/1 -> Add19/2
  Gain11/1 -> Add5/2
  Add20/1 -> Add21/2
  Constant15/1 -> Product11/1
  [e1] -> Product11/2
  Product11/1 -> Add21/3
  [dv5] -> Add18/1
  Add18/1 -> Add21/1
  [dvodi] -> Add18/2
  [dvodi] -> Add21/4
  [w15] -> Add3/1
  [w16] -> Add3/2
  Add3/1 -> Add11/3
  Neural Network 1/1(Sz1) -> [Sf]
  [vod5] -> Add6/1
  [vod] -> Add6/2
  Add6/1 -> Add14/3
  [S] -> Product8/1
  Constant7/1 -> Product8/2
  [e2] -> Product8/3
  Product8/1 -> Add9/1
  Constant8/1 -> Product10/1
  [W] -> Product10/2
  Product10/1 -> Add9/2
  Constant9/1 -> Product10/3
  Add9/1 -> Integrator2/1
  Integrator2/1 -> [W]
  [e2] -> Product10/4
  [Sf] -> Product13/1
  Constant12/1 -> Product13/2
  [ef] -> Product13/3
  Product13/1 -> Add12/1
  Constant13/1 -> Product12/1
  [Wf] -> Product12/2
  Product12/1 -> Add12/2
  Constant11/1 -> Product12/3
  Add12/1 -> Integrator3/1
  Integrator3/1 -> [Wf]
  [ef] -> Product12/4
  Gain5/1 -> Add14/1
  Neural Network 2/1(Sz1) -> [S]
  Constant4/1 -> Neural Network 2/2(mu)
  Mux2/1 -> Neural Network 2/1(X)
  Constant3/1 -> Neural Network 1/2(mu)
  Mux1/1 -> Neural Network 1/1(X)
  [ti] -> Switch4/2
  Add11/1 -> Switch4/1
  Switch4/1 -> [ef]
  [P] -> n/1
  Un3/1 -> Sum10/1  "f"
  Sum10/1 -> Add23/2
  n/1 -> [MP6], Sum10/2
  [w1] -> Add23/1
  Add23/1 -> Switch4/3
  Integrator4/1 -> [wt]
  Integrator1/1 -> [w1], f1/1, Integrator4/1
  Add7/1 -> Integrator1/1
  [ti] -> Switch2/2
  Add16/1 -> Switch2/3
  Add14/1 -> Switch2/1, [E6]
  Switch2/1 -> [e1]
  [vod] -> Add16/1
  [Q] -> m/1
  Un1/1 -> Sum11/2
  m/1 -> [NQ6], Sum11/1
  Sum11/1 -> Add16/2
  [ti] -> Switch3/2
  Switch3/1 -> [e2]
  Add21/1 -> Switch3/1
  Add17/1 -> Switch3/3
  [dvodi] -> Add17/2
  Constant17/1 -> Product16/1
  [e1] -> Product16/2
  Product16/1 -> Add17/1
  Constant18/1 -> Product17/1
  [NQ6] -> Product17/2
  Product17/1 -> Add22/1
  [Q66] -> Gain8/1
  Add22/1 -> Add17/3
  Gain8/1 -> Add22/2
  connections:
  C/RConn1 -- Ground1/LConn1 -- C/RConn3 -- C/RConn2
  L/RConn2 -- Three-Phase V-I Measurement1/LConn2 -- C/LConn2
  L/RConn1 -- Three-Phase V-I Measurement1/LConn1 -- C/LConn1
  L/RConn3 -- Three-Phase V-I Measurement1/LConn3 -- C/LConn3
  Controlled Voltage Source/LConn1 -- Controlled Voltage Source1/LConn1 -- Ground/LConn1 -- Controlled Voltage Source2/LConn1
  Three-Phase V-I Measurement/LConn1 -- Controlled Voltage Source/RConn1
  Controlled Voltage Source1/RConn1 -- Three-Phase V-I Measurement/LConn2
  Controlled Voltage Source2/RConn1 -- Three-Phase V-I Measurement/LConn3
  Three-Phase V-I Measurement/RConn1 -- L/LConn1
  Three-Phase V-I Measurement/RConn2 -- L/LConn2
  Three-Phase V-I Measurement/RConn3 -- L/LConn3
  Three-Phase Series RLC Branch4/RConn1 -- Three-Phase V-I Measurement1/RConn1
  Three-Phase Series RLC Branch4/RConn2 -- Three-Phase V-I Measurement1/RConn2
  Three-Phase Series RLC Branch4/RConn3 -- Three-Phase V-I Measurement1/RConn3
  Three-Phase Series RLC Branch4/LConn3 -- c/RConn1
  Three-Phase Series RLC Branch4/LConn2 -- b/RConn1
  Three-Phase Series RLC Branch4/LConn1 -- a/RConn1
